simulink model "BLDCctrlBasedOnMBDPILtop"  (R2020b)
settings: Solver=FixedStepDiscrete  StartTime=0.0  StopTime=inf  FixedStep=0.0001  RelTol=1e-3
settings Model: Creator=k  LastModifiedBy=k

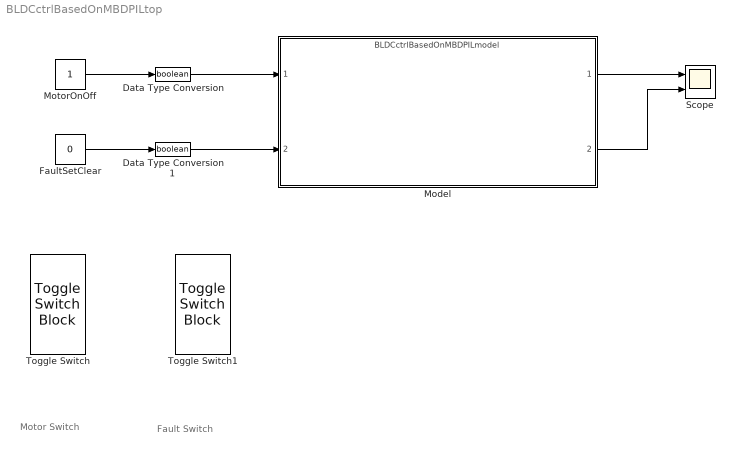
== system BLDCctrlBasedOnMBDPILtop ==
  note: Fault Switch
  note: Motor Switch
  Data Type Conversion : DataTypeConversion  OutDataTypeStr=boolean
  Data Type Conversion1 : DataTypeConversion  OutDataTypeStr=boolean
  FaultSetClear : Constant  Value=0
  Model : ModelReference  ModelNameDialog=BLDCctrlBasedOnMBDPILmodel.slx  SimulationMode=Processor-in-the-loop (PIL)  ModelReferenceVersion=1.28
  MotorOnOff : Constant
  Scope : Scope  NumInputPorts=2
  Toggle Switch : ToggleSwitchBlock  LabelPosition=Hide
      settings: Values={{'Off', 'On'}, [0 1]}
  Toggle Switch1 : ToggleSwitchBlock  LabelPosition=Hide
      settings: Values={{'Off', 'On'}, [0 1]}
  wires:
  Data Type Conversion/1 -> Model/1
  Data Type Conversion1/1 -> Model/2
  FaultSetClear/1 -> Data Type Conversion1/1
  MotorOnOff/1 -> Data Type Conversion/1
  Model/1 -> Scope/1
  Model/2 -> Scope/2
